simulink subsystem "PID"  (R2024a)
settings: Solver=VariableStepAuto  StartTime=0.0  StopTime=10.0  RelTol=1e-3
undefined symbols (not defined in the file or in its folder): controlRate, Kd, Ki, Kp, Tw
settings Model: Creator=Peter  LastModifiedBy=Peter

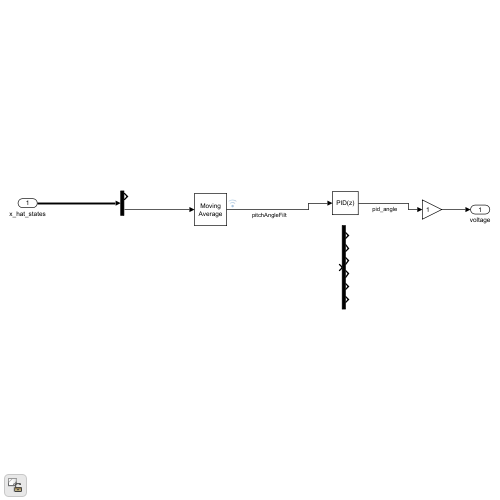
[thumbnail: Simulink's stored preview of the top-level diagram]
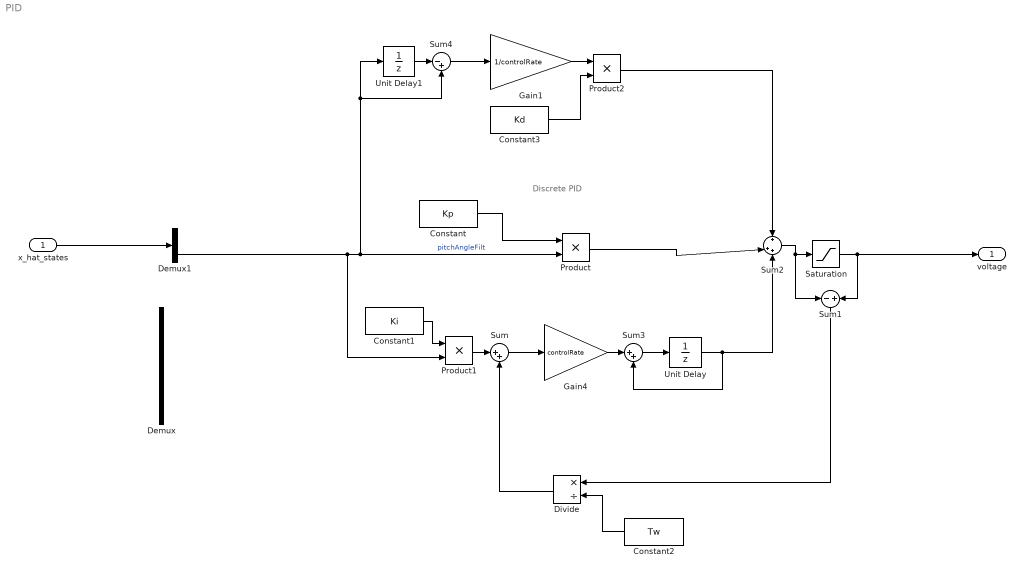
== system PID ==
  note: Discrete PID
  x_hat_states : Inport
  Constant : Constant  Value=Kp  OutDataTypeStr=single
  Constant1 : Constant  Value=Ki  OutDataTypeStr=single
  Constant2 : Constant  Value=Tw  OutDataTypeStr=single
  Constant3 : Constant  Value=Kd  OutDataTypeStr=single
  Demux : Demux  Outputs=6
  Demux1 : Demux  Outputs=2
  Divide : Product  Inputs=*/
  Gain1 : Gain  Gain=1/controlRate
  Gain4 : Gain  Gain=controlRate
  Product : Product
  Product1 : Product
  Product2 : Product
  Saturation : Saturate  UpperLimit=12  LowerLimit=-12
  Sum : Sum  Inputs=|++
  Sum1 : Sum  Inputs=-|+
  Sum2 : Sum  Inputs=+|++
  Sum3 : Sum  Inputs=|++
  Sum4 : Sum  Inputs=|-+
  Unit Delay : UnitDelay  SampleTime=-1  HasFrameUpgradeWarning=on
  Unit Delay1 : UnitDelay  SampleTime=-1  HasFrameUpgradeWarning=on
  voltage : Outport
  wires:
  x_hat_states/1 -> Demux1/1
  Saturation/1 -> voltage/1, Sum1/2
  Demux1/2 -> Product1/2, Product/2, Sum4/2, Unit Delay1/1  "pitchAngleFilt"
  Sum2/1 -> Sum1/1, Saturation/1
  Product/1 -> Sum2/2
  Product1/1 -> Sum/1
  Sum1/1 -> Divide/1
  Divide/1 -> Sum/2
  Sum/1 -> Gain4/1
  Sum3/1 -> Unit Delay/1
  Gain4/1 -> Sum3/1
  Unit Delay/1 -> Sum3/2, Sum2/3
  Constant/1 -> Product/1
  Constant1/1 -> Product1/1
  Constant2/1 -> Divide/2
  Unit Delay1/1 -> Sum4/1
  Sum4/1 -> Gain1/1
  Constant3/1 -> Product2/2
  Gain1/1 -> Product2/1
  Product2/1 -> Sum2/1
